simulink model "SRManCw5_ZADANIE2_MODEL"  (R2018a)
settings: Solver=ode45  StartTime=0.0  StopTime=tend  MaxStep=Tp  RelTol=1e-3
values from neighbouring files (symbols this model uses):
  Delta = diag([delta delta])    [SRManCw5_ZADANIE2_SKRYPT.m]
  delta = 5000.0    (= 5000)    [SRManCw5_ZADANIE2_SKRYPT.m]
  initConditionsPos = [0; 0]    [SRManCw5_ZADANIE2_SKRYPT.m]
  initConditionsVel = [0; 0]    [SRManCw5_ZADANIE2_SKRYPT.m]
  Kv = Mhat * s    [SRManCw5_ZADANIE2_KV.m]    (also in SRManCw5_ZADANIE2_SKRYPT.m = diag([w w]))
  Lambda = diag([k k])    [SRManCw5_ZADANIE2_SKRYPT.m]
  Mhat = [m11 m12; m21 m22]    [SRManCw5_ESTYMATA_MACIERZY_MxQrDotDot.m]    (also in SRManCw5_ZADANIE2_KV.m = [m1 m2; m3 m4])
  omega1 = 0.6    [SRManCw5_ZADANIE2_SKRYPT.m]
  omega2 = 0.7    [SRManCw5_ZADANIE2_SKRYPT.m]
  phatInitConditions = [0.1 0.1 0.1 0.1 0.1 0.1 0.1]    [SRManCw5_ZADANIE2_SKRYPT.m]
  Qd01 = 0.0025    [SRManCw5_ZADANIE2_SKRYPT.m]
  Qd02 = 0.0025    [SRManCw5_ZADANIE2_SKRYPT.m]
  Qd1 = 1    [SRManCw5_ZADANIE2_SKRYPT.m]
  Qd11 = 0.0020    (= 0.002)    [SRManCw5_ZADANIE2_SKRYPT.m]
  Qd12 = 0.002    [SRManCw5_ZADANIE2_SKRYPT.m]
  Qd1const = 1    [SRManCw5_ZADANIE2_SKRYPT.m]
  Qd2 = 1    [SRManCw5_ZADANIE2_SKRYPT.m]
  Qd21 = 0.0015    [SRManCw5_ZADANIE2_SKRYPT.m]
  Qd22 = 0.0015    [SRManCw5_ZADANIE2_SKRYPT.m]
  Qd2const = 1    [SRManCw5_ZADANIE2_SKRYPT.m]
  Qd31 = 0.001    [SRManCw5_ZADANIE2_SKRYPT.m]
  Qd32 = 0.001    [SRManCw5_ZADANIE2_SKRYPT.m]
libraries: dsppolyfun x6, simulink x2
settings Model: Creator=szymon  LastModifiedBy=szymon

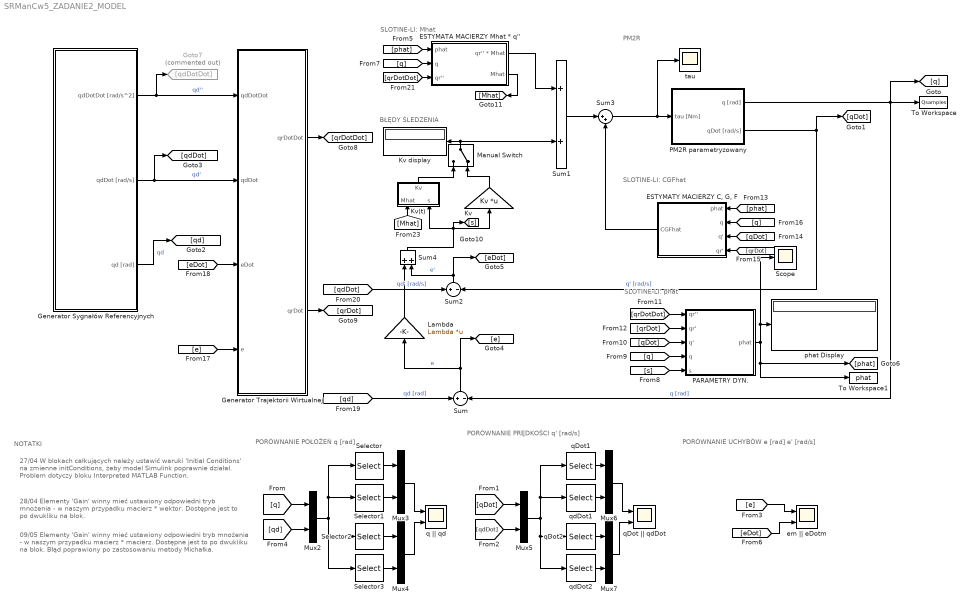
== system SRManCw5_ZADANIE2_MODEL ==
  note: SLOTINE-LI: CGFhat
  note: NOTATKI
  note: 27/04 W blokach całkujących należy ustawić waruki
      | 'Initial Conditions' na zmienne initConditions, żeby model
      | Simulink poprawnie działał. Problem dotyczy bloku
      | Interpreted MATLAB Function.
  note: 28/04 Elementy 'Gain' winny mieć ustawiony odpowiedni tryb
      | mnożenia - w naszym przypadku macierz * wektor.
      | Dostępne jest to po dwukliku na blok.
  note: 09/05 Elementy 'Gain' winny mieć ustawiony odpowiedni tryb
      | mnożenia - w naszym przypadku macierz * macierz.
      | Dostępne jest to po dwukliku na blok. Błąd poprawiony po
      | zastosowaniu metody Michałka.
  note: PM2R
  note: PORÓWNANIE POŁOŻEŃ
      | q [rad]
  note: PORÓWNANIE UCHYBÓW
      | e  [rad]
      | e' [rad/s]
  note: PORÓWNANIE PRĘDKOŚCI
      | q' [rad/s]
  note: SLOTINE-LI: Mhat
  note: SLOTINE-LI: phat
  note: BŁĘDY ŚLEDZENIA
  ESTYMATA MACIERZY Mhat * q'' : Subsystem
  "ESTYMATY MACIERZY C, G, F" : Subsystem
  Generator Trajektorii Wirtualnej : Subsystem
  Generator Sygnałów Referencyjnych : Subsystem
  Goto7 : Goto  Commented=on  GotoTag=qdDotDot
  Kv : Gain  Gain=Kv  Multiplication=Matrix(K*u) (u vector)
  Kv display : Display
  Kv(t) : Subsystem
  Lambda : Gain  Gain=Lambda  Multiplication=Matrix(K*u) (u vector)
  Manual Switch : ManualSwitch  CurrentSetting=0
  Mux{2..7} (6 alike) : Mux  Inputs=2
  PARAMETRY DYN. : Subsystem
  PM2R parametryzowany : Subsystem
  Scope : Scope
  Selector : Selector  InputPortWidth=4  IndexOptions=Index vector (dialog)  Indices=[1]  OutputSizes=1
  Selector1 : Selector  InputPortWidth=4  IndexOptions=Index vector (dialog)  Indices=[3]  OutputSizes=1
  Selector2 : Selector  InputPortWidth=4  IndexOptions=Index vector (dialog)  Indices=[2]  OutputSizes=1
  Selector3 : Selector  InputPortWidth=4  IndexOptions=Index vector (dialog)  Indices=[4]  OutputSizes=1
  Sum : Sum  Inputs=+-
  Sum1 : Sum
  Sum2 : Sum  Inputs=+-
  Sum3 : Sum  Inputs=|++
  Sum4 : Sum
  To Workspace : ToWorkspace  VariableName=Qsamples  SampleTime=-1
  To Workspace1 : ToWorkspace  VariableName=phat  SampleTime=-1
      settings: MaxDataPoints=1
  em || eDotm : Scope  NumInputPorts=2
  phat Display : Display
  q || qd : Scope  NumInputPorts=2
  qDot || qdDot : Scope  NumInputPorts=2
  qDot1 : Selector  InputPortWidth=4  IndexOptions=Index vector (dialog)  Indices=[1]  OutputSizes=1
  qDot2 : Selector  InputPortWidth=4  IndexOptions=Index vector (dialog)  Indices=[2]  OutputSizes=1
  qdDot1 : Selector  InputPortWidth=4  IndexOptions=Index vector (dialog)  Indices=[3]  OutputSizes=1
  qdDot2 : Selector  InputPortWidth=4  IndexOptions=Index vector (dialog)  Indices=[4]  OutputSizes=1
  tau : Scope
  wires:
  Sum2/1 -> [eDot], Sum4/2  "e'"
  Manual Switch/1 -> Kv display/1, Sum1/2
  Sum/1 -> Lambda/1, [e]  "e"
  Sum1/1 -> Sum3/1
  Sum3/1 -> tau/1, PM2R parametryzowany/1(tau [Nm])
  "ESTYMATY MACIERZY C, G, F"/1(CGFhat) -> Sum3/2
  [phat] -> ESTYMATA MACIERZY Mhat * q''/1(phat)
  [q] -> ESTYMATA MACIERZY Mhat * q''/2(q)
  ESTYMATA MACIERZY Mhat * q''/1(qr'' * Mhat) -> Sum1/1
  [s] -> PARAMETRY DYN./5(s)
  [q] -> PARAMETRY DYN./4(q)
  [qDot] -> PARAMETRY DYN./3(q')
  [qrDot] -> PARAMETRY DYN./2(qr')
  [qrDotDot] -> PARAMETRY DYN./1(qr'')
  [phat] -> "ESTYMATY MACIERZY C, G, F"/1(phat)
  [qrDot] -> "ESTYMATY MACIERZY C, G, F"/4(qr')
  [qDot] -> "ESTYMATY MACIERZY C, G, F"/3(q')
  [q] -> "ESTYMATY MACIERZY C, G, F"/2(q)
  PM2R parametryzowany/2(qDot [rad/s]) -> Sum2/2, [qDot]  "q' [rad/s]"
  PM2R parametryzowany/1(q [rad]) -> [q], To Workspace/1, Sum/2  "q [rad]"
  [qDot] -> Mux5/1
  Selector/1 -> Mux3/1
  [q] -> Mux2/1
  Selector2/1 -> Mux4/1
  qdDot1/1 -> Mux6/2
  Selector3/1 -> Mux4/2
  Mux2/1 -> Selector3/1, Selector2/1, Selector1/1, Selector/1
  qDot2/1 -> Mux7/1
  [eDot] -> em || eDotm/2
  qdDot2/1 -> Mux7/2
  [e] -> em || eDotm/1
  Mux4/1 -> q || qd/2
  Mux5/1 -> qdDot2/1, qDot2/1, qdDot1/1, qDot1/1
  [qdDot] -> Mux5/2
  qDot1/1 -> Mux6/1
  Selector1/1 -> Mux3/2
  Mux7/1 -> qDot || qdDot/2
  Mux3/1 -> q || qd/1
  Mux6/1 -> qDot || qdDot/1
  [qd] -> Mux2/2
  [e] -> Generator Trajektorii Wirtualnej/4(e)
  [eDot] -> Generator Trajektorii Wirtualnej/3(eDot)
  Generator Sygnałów Referencyjnych/1(qdDotDot [rad/s^2]) -> Goto7/1, Generator Trajektorii Wirtualnej/1(qdDotDot)  "qd''"
  Generator Trajektorii Wirtualnej/1(qrDotDot) -> [qrDotDot]
  Generator Sygnałów Referencyjnych/2(qdDot [rad/s]) -> [qdDot], Generator Trajektorii Wirtualnej/2(qdDot)  "qd'"
  Generator Sygnałów Referencyjnych/3(qd [rad]) -> [qd]  "qd"
  [qd] -> Sum/1  "qd [rad]"
  [qdDot] -> Sum2/1  "qd' [rad/s]"
  Generator Trajektorii Wirtualnej/2(qrDot) -> [qrDot]
  Lambda/1 -> Sum4/1
  Sum4/1 -> [s], Kv/1, Kv(t)/2(s)
  [qrDotDot] -> ESTYMATA MACIERZY Mhat * q''/3("qr'' ")
  PARAMETRY DYN./1(phat) -> To Workspace1/1, [phat], Scope/1, phat Display/1
  Kv/1 -> Manual Switch/2
  ESTYMATA MACIERZY Mhat * q''/2(Mhat) -> [Mhat]
  Kv(t)/1(Kv) -> Manual Switch/1
  [Mhat] -> Kv(t)/1(Mhat)

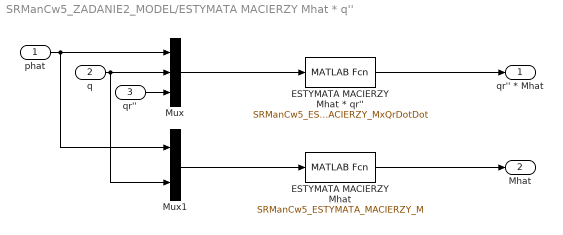
== system SRManCw5_ZADANIE2_MODEL/ESTYMATA MACIERZY Mhat * q'' ==
  phat : Inport
  q : Inport  Port=2
  "qr'' " : Inport  Port=3
  ESTYMATA MACIERZY Mhat : MATLABFcn  MATLABFcn=SRManCw5_ESTYMATA_MACIERZY_M
  ESTYMATA MACIERZY Mhat * qr'' : MATLABFcn  MATLABFcn=SRManCw5_ESTYMATA_MACIERZY_MxQrDotDot
  Mux : Mux  Inputs=3
  Mux1 : Mux  Inputs=2
  qr'' * Mhat : Outport
  Mhat : Outport  Port=2
  wires:
  ESTYMATA MACIERZY Mhat * qr''/1 -> qr'' * Mhat/1
  Mux/1 -> ESTYMATA MACIERZY Mhat * qr''/1
  phat/1 -> Mux1/1, Mux/1
  q/1 -> Mux1/2, Mux/2
  "qr'' "/1 -> Mux/3
  ESTYMATA MACIERZY Mhat/1 -> Mhat/1
  Mux1/1 -> ESTYMATA MACIERZY Mhat/1

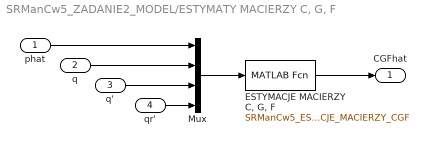
== system SRManCw5_ZADANIE2_MODEL/ESTYMATY MACIERZY C, G, F ==
  phat : Inport
  q : Inport  Port=2
  q' : Inport  Port=3
  qr' : Inport  Port=4
  "ESTYMACJE MACIERZY C, G, F" : MATLABFcn  MATLABFcn=SRManCw5_ESTYMACJE_MACIERZY_CGF
  Mux : Mux
  CGFhat : Outport
  wires:
  "ESTYMACJE MACIERZY C, G, F"/1 -> CGFhat/1
  Mux/1 -> "ESTYMACJE MACIERZY C, G, F"/1
  q/1 -> Mux/2
  q'/1 -> Mux/3
  qr'/1 -> Mux/4
  phat/1 -> Mux/1

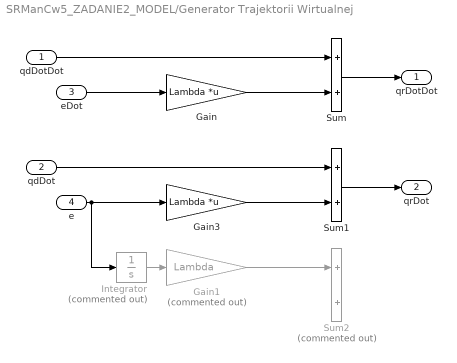
== system SRManCw5_ZADANIE2_MODEL/Generator Trajektorii Wirtualnej ==
  qdDotDot : Inport
  qdDot : Inport  Port=2
  eDot : Inport  Port=3
  e : Inport  Port=4
  Gain : Gain  Gain=Lambda  Multiplication=Matrix(K*u) (u vector)
  Gain1 : Gain  Commented=on  Gain=Lambda
  Gain3 : Gain  Gain=Lambda  Multiplication=Matrix(K*u) (u vector)
  Integrator : Integrator  Commented=on
  Sum : Sum
  Sum1 : Sum
  Sum2 : Sum  Commented=on
  qrDotDot : Outport
  qrDot : Outport  Port=2
  wires:
  qdDotDot/1 -> Sum/1
  eDot/1 -> Gain/1
  Gain/1 -> Sum/2
  Sum/1 -> qrDotDot/1
  Sum1/1 -> qrDot/1
  qdDot/1 -> Sum1/1
  Gain3/1 -> Sum1/2
  e/1 -> Integrator/1, Gain3/1
  Integrator/1 -> Gain1/1
  Gain1/1 -> Sum2/1

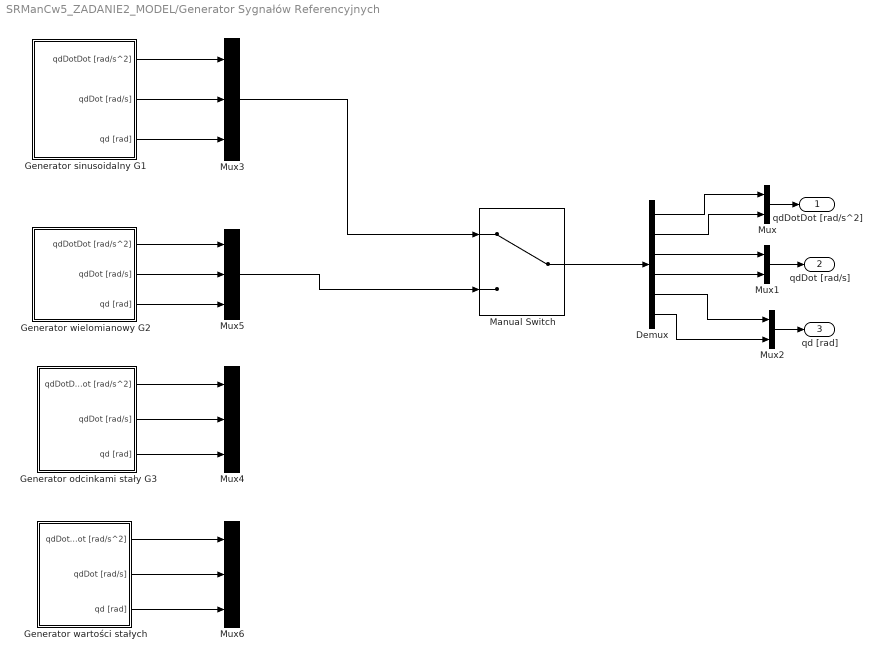
== system SRManCw5_ZADANIE2_MODEL/Generator Sygnałów Referencyjnych ==
  Demux : Demux  Outputs=6
  "Generator odcinkami stały G3 " : Subsystem
  Generator sinusoidalny G1 : Subsystem
  Generator wielomianowy G2 : Subsystem
  Generator wartości stałych : Subsystem
  Manual Switch : ManualSwitch
  Mux : Mux  Inputs=2
  Mux1 : Mux  Inputs=2
  Mux2 : Mux  Inputs=2
  Mux{3..6} (4 alike) : Mux  Inputs=3
  qdDotDot [rad/s^2] : Outport
  qdDot [rad/s] : Outport  Port=2
  qd [rad] : Outport  Port=3
  wires:
  Mux/1 -> qdDotDot [rad/s^2]/1
  Mux2/1 -> qd [rad]/1
  Mux1/1 -> qdDot [rad/s]/1
  Demux/1 -> Mux/1
  Demux/2 -> Mux/2
  Demux/3 -> Mux1/1
  Demux/4 -> Mux1/2
  Demux/5 -> Mux2/1
  Demux/6 -> Mux2/2
  Generator sinusoidalny G1/2(qdDot [rad/s]) -> Mux3/2
  Generator sinusoidalny G1/1(qdDotDot [rad/s^2]) -> Mux3/1
  Generator sinusoidalny G1/3(qd [rad]) -> Mux3/3
  "Generator odcinkami stały G3 "/1(qdDotDot [rad/s^2]) -> Mux4/1
  "Generator odcinkami stały G3 "/2(qdDot [rad/s]) -> Mux4/2
  "Generator odcinkami stały G3 "/3(qd [rad]) -> Mux4/3
  Generator wielomianowy G2/1(qdDotDot [rad/s^2]) -> Mux5/1
  Generator wielomianowy G2/2(qdDot [rad/s]) -> Mux5/2
  Generator wielomianowy G2/3(qd [rad]) -> Mux5/3
  Generator wartości stałych/1(qdDotDot [rad/s^2]) -> Mux6/1
  Generator wartości stałych/3(qd [rad]) -> Mux6/3
  Generator wartości stałych/2(qdDot [rad/s]) -> Mux6/2
  Manual Switch/1 -> Demux/1
  Mux3/1 -> Manual Switch/1
  Mux5/1 -> Manual Switch/2

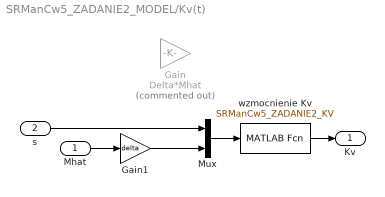
== system SRManCw5_ZADANIE2_MODEL/Kv(t) ==
  Mhat : Inport
  s : Inport  Port=2
  Gain : Gain  Commented=on  Gain=Delta*Mhat
  Gain1 : Gain  Gain=delta
  Mux : Mux  Inputs=2
  wzmocnienie Kv : MATLABFcn  MATLABFcn=SRManCw5_ZADANIE2_KV
  Kv : Outport
  wires:
  s/1 -> Mux/1
  wzmocnienie Kv/1 -> Kv/1
  Mux/1 -> wzmocnienie Kv/1
  Mhat/1 -> Gain1/1
  Gain1/1 -> Mux/2

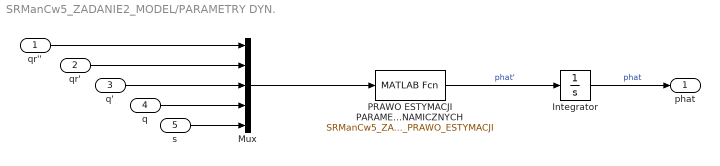
== system SRManCw5_ZADANIE2_MODEL/PARAMETRY DYN. ==
  qr'' : Inport
  qr' : Inport  Port=2
  q' : Inport  Port=3
  q : Inport  Port=4
  s : Inport  Port=5
  Integrator : Integrator  InitialCondition=phatInitConditions
  Mux : Mux  Inputs=5
  PRAWO ESTYMACJI PARAMETRÓW DYNAMICZNYCH : MATLABFcn  MATLABFcn=SRManCw5_ZADANIE2_PRAWO_ESTYMACJI
  phat : Outport
  wires:
  Mux/1 -> PRAWO ESTYMACJI PARAMETRÓW DYNAMICZNYCH/1
  qr'/1 -> Mux/2
  qr''/1 -> Mux/1
  PRAWO ESTYMACJI PARAMETRÓW DYNAMICZNYCH/1 -> Integrator/1  "phat'"
  q'/1 -> Mux/3
  q/1 -> Mux/4
  Integrator/1 -> phat/1  "phat"
  s/1 -> Mux/5

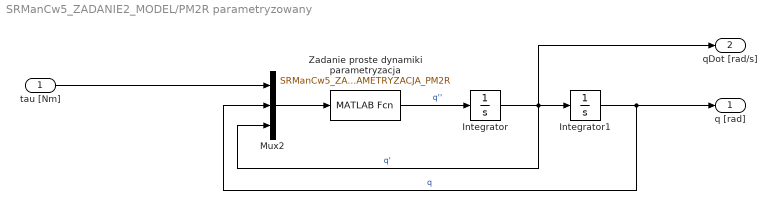
== system SRManCw5_ZADANIE2_MODEL/PM2R parametryzowany ==
  tau [Nm] : Inport
  Integrator : Integrator  InitialCondition=initConditionsVel
  Integrator1 : Integrator  InitialCondition=initConditionsPos
  Mux2 : Mux  Inputs=3
  Zadanie proste dynamiki parametryzacja : MATLABFcn  MATLABFcn=SRManCw5_ZADANIE2_PARAMETRYZACJA_PM2R  Output1D=off
  q [rad] : Outport
  qDot [rad/s] : Outport  Port=2
  wires:
  Mux2/1 -> Zadanie proste dynamiki parametryzacja/1
  Integrator1/1 -> q [rad]/1, Mux2/2  "q"
  Integrator/1 -> qDot [rad/s]/1, Mux2/3, Integrator1/1  "q'"
  tau [Nm]/1 -> Mux2/1
  Zadanie proste dynamiki parametryzacja/1 -> Integrator/1  "q''"

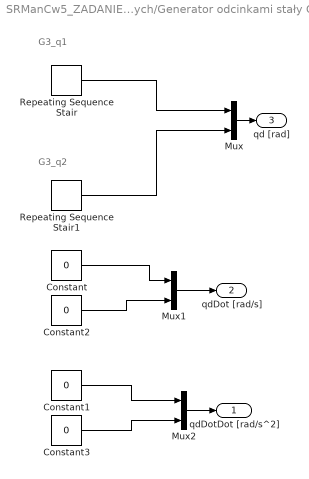
== system SRManCw5_ZADANIE2_MODEL/Generator Sygnałów Referencyjnych/Generator odcinkami stały G3  ==
  note: G3_q2
  note: G3_q1
  Constant{,1..3} (4 alike) : Constant  Value=0
  Mux : Mux  Inputs=2
  Mux1 : Mux  Inputs=2
  Mux2 : Mux  Inputs=2
  Repeating Sequence Stair : simulink/Sources/Repeating Sequence Stair  OutValues=[Qd1const 0].'  tsamp=Ta  OutMin=[]  OutMax=[]  OutDataTypeStr=double  OutputDataTypeScalingMode=double  OutDataType=fixdt(0,8)  ConRadixGroup=Best Precision: Vector-wise  OutScaling=2^-12
  Repeating Sequence Stair1 : simulink/Sources/Repeating Sequence Stair  OutValues=[Qd2const 0 ].'  tsamp=Tb  OutMin=[]  OutMax=[]  OutDataTypeStr=double  OutputDataTypeScalingMode=double  OutDataType=fixdt(0,8)  ConRadixGroup=Best Precision: Vector-wise  OutScaling=2^-12
  qdDotDot [rad/s^2] : Outport
  qdDot [rad/s] : Outport  Port=2
  qd [rad] : Outport  Port=3
  wires:
  Constant/1 -> Mux1/1
  Repeating Sequence Stair1/1 -> Mux/2
  Repeating Sequence Stair/1 -> Mux/1
  Mux/1 -> qd [rad]/1
  Constant1/1 -> Mux2/1
  Constant2/1 -> Mux1/2
  Constant3/1 -> Mux2/2
  Mux2/1 -> qdDotDot [rad/s^2]/1
  Mux1/1 -> qdDot [rad/s]/1

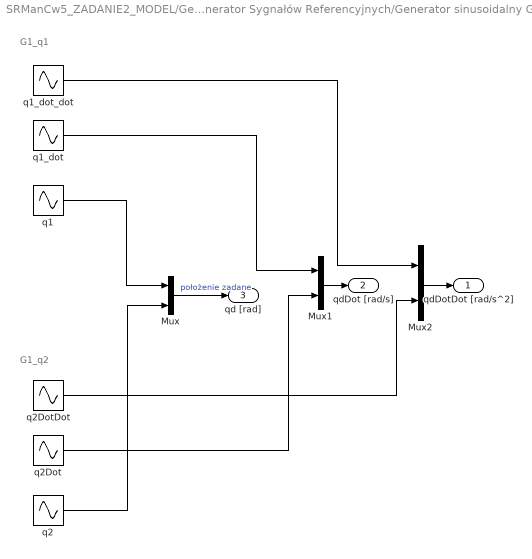
== system SRManCw5_ZADANIE2_MODEL/Generator Sygnałów Referencyjnych/Generator sinusoidalny G1 ==
  note: G1_q1
  note: G1_q2
  Mux : Mux  Inputs=2
  Mux1 : Mux  Inputs=2
  Mux2 : Mux  Inputs=2
  "q1 " : Sin  Amplitude=Qd1  Frequency=omega1  SampleTime=0
  q1_dot : Sin  Amplitude=omega1*Qd1  Frequency=omega1  Phase=pi/2  SampleTime=0
  "q1_dot_dot " : Sin  Amplitude=-omega1^2*Qd1  Frequency=omega1  SampleTime=0
  q2 : Sin  Amplitude=Qd2  Frequency=omega2  SampleTime=0
  q2Dot : Sin  Amplitude=omega2*Qd2  Frequency=omega2  Phase=pi/2  SampleTime=0
  "q2DotDot " : Sin  Amplitude=-omega2^2*Qd2  Frequency=omega2  SampleTime=0
  qdDotDot [rad/s^2] : Outport
  qdDot [rad/s] : Outport  Port=2
  qd [rad] : Outport  Port=3
  wires:
  Mux1/1 -> qdDot [rad/s]/1
  Mux2/1 -> qdDotDot [rad/s^2]/1
  q2/1 -> Mux/2
  "q1 "/1 -> Mux/1
  Mux/1 -> qd [rad]/1  "położenie zadane"
  "q1_dot_dot "/1 -> Mux2/1
  q1_dot/1 -> Mux1/1
  "q2DotDot "/1 -> Mux2/2
  q2Dot/1 -> Mux1/2

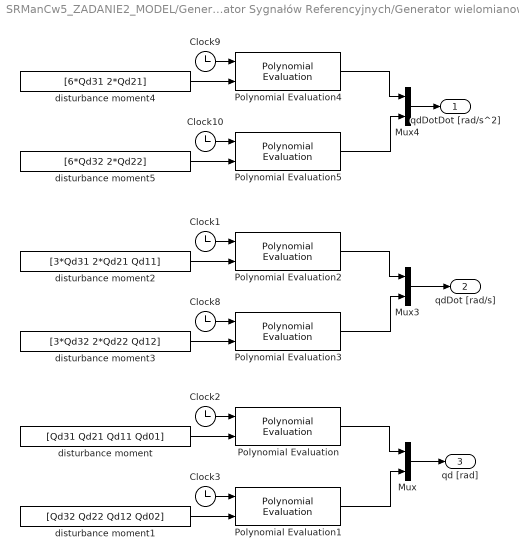
== system SRManCw5_ZADANIE2_MODEL/Generator Sygnałów Referencyjnych/Generator wielomianowy G2 ==
  Clock{1..3,8..10} (6 alike) : Clock
  Mux : Mux  Inputs=2
  Mux3 : Mux  Inputs=2
  Mux4 : Mux  Inputs=2
  Polynomial Evaluation{,1..5} (6 alike) : dsppolyfun/Polynomial Evaluation  useConstCoeffs=off  constCoeffs=[5 4 3 2 1]
      settings: SourceProductName=DSP System Toolbox  SourceProductBaseCode=DS
  disturbance moment : Constant  Value=[Qd31 Qd21 Qd11 Qd01]
  disturbance moment1 : Constant  Value=[Qd32 Qd22 Qd12 Qd02]
  disturbance moment2 : Constant  Value=[3*Qd31 2*Qd21 Qd11]
  disturbance moment3 : Constant  Value=[3*Qd32 2*Qd22 Qd12]
  disturbance moment4 : Constant  Value=[6*Qd31 2*Qd21]
  disturbance moment5 : Constant  Value=[6*Qd32 2*Qd22]
  qdDotDot [rad/s^2] : Outport
  qdDot [rad/s] : Outport  Port=2
  qd [rad] : Outport  Port=3
  wires:
  Mux/1 -> qd [rad]/1
  disturbance moment/1 -> Polynomial Evaluation/2
  disturbance moment1/1 -> Polynomial Evaluation1/2
  Polynomial Evaluation/1 -> Mux/1
  Polynomial Evaluation1/1 -> Mux/2
  Clock2/1 -> Polynomial Evaluation/1
  Clock3/1 -> Polynomial Evaluation1/1
  Mux3/1 -> qdDot [rad/s]/1
  Clock1/1 -> Polynomial Evaluation2/1
  disturbance moment3/1 -> Polynomial Evaluation3/2
  Polynomial Evaluation2/1 -> Mux3/1
  disturbance moment2/1 -> Polynomial Evaluation2/2
  Polynomial Evaluation3/1 -> Mux3/2
  Clock8/1 -> Polynomial Evaluation3/1
  Clock10/1 -> Polynomial Evaluation5/1
  Polynomial Evaluation5/1 -> Mux4/2
  Polynomial Evaluation4/1 -> Mux4/1
  disturbance moment5/1 -> Polynomial Evaluation5/2
  Clock9/1 -> Polynomial Evaluation4/1
  disturbance moment4/1 -> Polynomial Evaluation4/2
  Mux4/1 -> qdDotDot [rad/s^2]/1

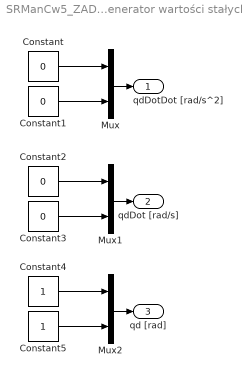
== system SRManCw5_ZADANIE2_MODEL/Generator Sygnałów Referencyjnych/Generator wartości stałych ==
  Constant{,1..3} (4 alike) : Constant  Value=0
  Constant4 : Constant
  Constant5 : Constant
  Mux : Mux  Inputs=2
  Mux1 : Mux  Inputs=2
  Mux2 : Mux  Inputs=2
  qdDotDot [rad/s^2] : Outport
  qdDot [rad/s] : Outport  Port=2
  qd [rad] : Outport  Port=3
  wires:
  Constant/1 -> Mux/1
  Mux/1 -> qdDotDot [rad/s^2]/1
  Constant1/1 -> Mux/2
  Constant2/1 -> Mux1/1
  Constant3/1 -> Mux1/2
  Mux1/1 -> qdDot [rad/s]/1
  Constant4/1 -> Mux2/1
  Constant5/1 -> Mux2/2
  Mux2/1 -> qd [rad]/1
